simulink model "bh_smd_COMP_MDL"  (R2018a)
settings: Solver=ode4  StartTime=0.0  StopTime=10.0  FixedStep=0.01  RelTol=1e-7
undefined symbols (not defined in the file): c, k, m, x_init, xdot_init
settings Model: Creator=bhorton  LastModifiedBy=bhorton
settings CodeAppCC: StateflowObjectComments=on

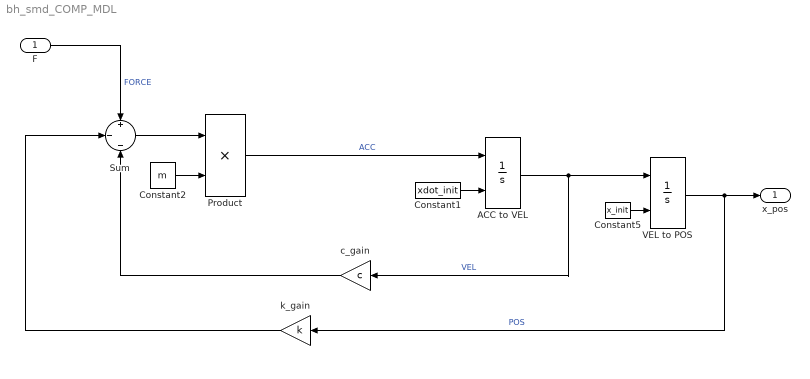
== system bh_smd_COMP_MDL ==
  F : Inport
  ACC to VEL : Integrator  InitialConditionSource=external
  Constant1 : Constant  Value=xdot_init
  Constant2 : Constant  Value=m
  Constant5 : Constant  Value=x_init
  Product : Product
  Sum : Sum  Inputs=+|-|-
  VEL to POS : Integrator  InitialConditionSource=external
  c_gain : Gain  Gain=c
  k_gain : Gain  Gain=k
  x_pos : Outport
  wires:
  F/1 -> Sum/1  "FORCE"
  Product/1 -> ACC to VEL/1  "ACC"
  ACC to VEL/1 -> c_gain/1, VEL to POS/1  "VEL"
  VEL to POS/1 -> x_pos/1, k_gain/1  "POS"
  Constant2/1 -> Product/2
  Constant1/1 -> ACC to VEL/2
  Constant5/1 -> VEL to POS/2
  Sum/1 -> Product/1
  c_gain/1 -> Sum/3
  k_gain/1 -> Sum/2
